simulink model "ErdMondBahn"  (R2014b)
settings: Solver=ode45  StartTime=0.0  StopTime=840000  RelTol=1e-3
libraries: simulink x1
settings Model: Creator=Florian  LastModifiedBy=Florian

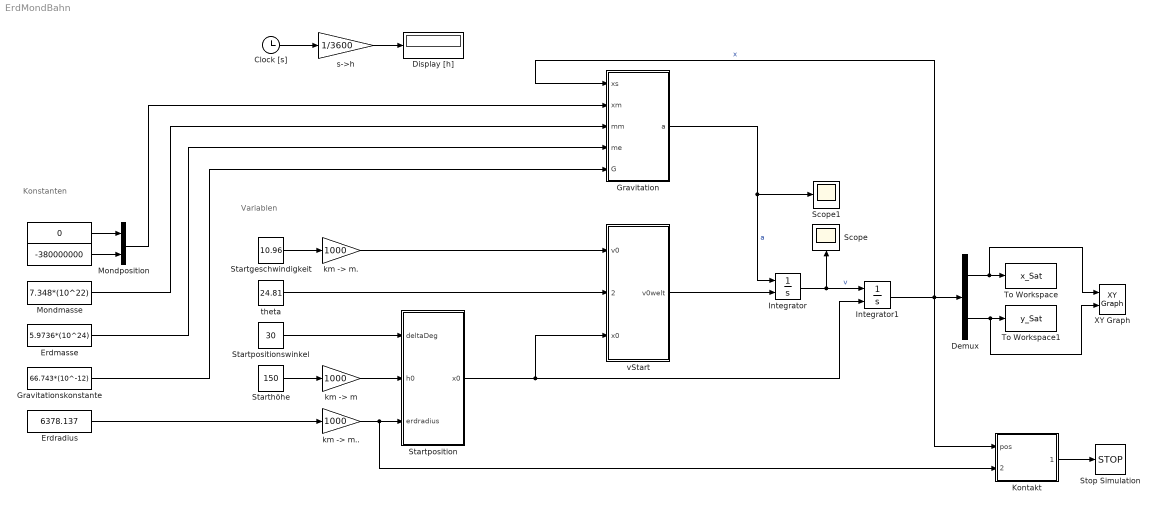
== system ErdMondBahn ==
  note: Konstanten
  note: Variablen
  "  " : Constant  Value=0
  "        " : Constant  Value=-380000000
  Clock [s] : Clock
  Demux : Demux  Outputs=2
  Display [h] : Display
  Erdmasse : Constant  Value=5.9736*(10^24)
  Erdradius : Constant  Value=6378.137
  Gravitation : MATLAB Function  TreatAsAtomicUnit=on
  Gravitationskonstante : Constant  Value=66.743*(10^-12)
  Integrator : Integrator  InitialConditionSource=external
  Integrator1 : Integrator  InitialConditionSource=external
  Kontakt : MATLAB Function  TreatAsAtomicUnit=on
  Mondmasse : Constant  Value=7.348*(10^22)
  Mondposition : Concatenate
  Scope : Scope
  Scope1 : Scope
  Startgeschwindigkeit : Constant  Value=10.96
  Starthöhe : Constant  Value=150
  Startposition : MATLAB Function  TreatAsAtomicUnit=on
  Startpositionswinkel : Constant  Value=30
  Stop Simulation : Stop
  To Workspace : ToWorkspace  VariableName=x_Sat  SampleTime=-1
  To Workspace1 : ToWorkspace  VariableName=y_Sat  SampleTime=-1
  XY Graph : simulink/Sinks/XY Graph  xmin=-22811188  xmax=22811188  ymin=-22811188  ymax=22811188  st=-1
  "km -> m" : Gain  Gain=1000
  "km -> m." : Gain  Gain=1000
  "km -> m.." : Gain  Gain=1000
  s->h : Gain  Gain=1/3600
  theta : Constant  Value=24.81
  vStart : MATLAB Function  TreatAsAtomicUnit=on
  wires:
  Erdradius/1 -> "km -> m.."/1
  Starthöhe/1 -> "km -> m"/1
  Startpositionswinkel/1 -> Startposition/1(deltaDeg)
  theta/1 -> vStart/2(thetaDeg)
  Startposition/1(x0) -> vStart/3(x0), Integrator1/2
  Kontakt/1(hasContact) -> Stop Simulation/1
  Clock [s]/1 -> s->h/1
  s->h/1 -> Display [h]/1
  Demux/1 -> XY Graph/1, To Workspace/1
  "km -> m"/1 -> Startposition/2(h0)
  "km -> m.."/1 -> Kontakt/2(erdradius), Startposition/3(erdradius)
  "km -> m."/1 -> vStart/1(v0)
  Gravitation/1(a) -> Integrator/1, Scope1/1  "a"
  Integrator/1 -> Integrator1/1, Scope/1  "v"
  Integrator1/1 -> Demux/1, Kontakt/1(pos), Gravitation/1(xs)  "x"
  Demux/2 -> XY Graph/2, To Workspace1/1
  Erdmasse/1 -> Gravitation/4(me)
  Gravitationskonstante/1 -> Gravitation/5(G)
  vStart/1(v0welt) -> Integrator/2
  Startgeschwindigkeit/1 -> "km -> m."/1
  Mondmasse/1 -> Gravitation/3(mm)
  "  "/1 -> Mondposition/1
  "        "/1 -> Mondposition/2
  Mondposition/1 -> Gravitation/2(xm)

== matlab function ErdMondBahn/vStart ==
  data: v0 input; thetaDeg input; x0 input; v0welt output
function v0welt = fcn(v0, thetaDeg, x0)
%-------------------------------------------------------------------------------------------------------
%Geben Sie eine EM-Funktion „vStart“ an,
%die aus den Parametern v0 ,  und der berechneten Startposition x0
%den Startgeschwindigkeitsvektor v0,Welt berechnet ( Anfangswert der Geschwindkt. in Weltkoordinaten).
%   Hinweis: - Einheitsvektoren in Tangential- und Normalenrichtung (n, t) aus x0 konstruieren,
%   - Tangential- und Normalkomponente der Startgeschwindigkeit (vt, vn) berechnen,
%   - aus n, t und (vt, vn) die Startgeschwindigkeit v0,Welt zusammenbauen.
%------------------------------------------------------------------------------------------------------


%Einheitsvektor von X0 (Normalenrichtung)
normalenrichtungX0 = x0 / norm(x0); %norm = Betrag -> x0/|x0|
%(Tangentialrichtung)
tangentialrichtungX0 = [normalenrichtungX0(2) ; -normalenrichtungX0(1)];  % [+;-]= im Uhrzeigersinn ; [-;+] = gegen Uhrzeigersinn


%Grad -> Bogenmaß
thetaBog = thetaDeg * (pi()/180);
%Tangential- und Normalkomponente der Startgeschwindigkeit
vt = cos(thetaBog) * v0;
vn = sin(thetaBog) * v0;


%Startgeschwindigkeit
v0welt = (norm(vt) * tangentialrichtungX0) + (norm(vn) * normalenrichtungX0);

== matlab function ErdMondBahn/Startposition ==
  data: deltaDeg input; x0 output; h0 input; erdradius input
function x0 = fcn(deltaDeg, h0, erdradius)
%-------------------------------------------------------------------------------------------------------
%Geben Sie eine Embedded-Matlab-(EM)-Funktion „Startposition“ an,
%die aus den Parametern delta(°), der Starthöhe h0 (km) sowie der Konstante „Erdradius“
%die Startposition x0 berechnet ( Anfangswert für die Position).
%------------------------------------------------------------------------------------------------------

%Grad -> Bogenmaß
deltaBog = deltaDeg* pi()/180;

hoehe = erdradius + h0;

x = cos(deltaBog)*(hoehe);
y = sin(deltaBog)*(hoehe);

x0 = [x;y];

== matlab function ErdMondBahn/Gravitation ==
  data: xs input; xm input; mm input; me input; a output; G input
function a = fcn(xs, xm, mm, me, G)
%-------------------------------------------------------------------------------------------------------
%Geben Sie eine EM-Funktion „Gravitation“ an,
%die aus der aktuellen Satellitenposition x,
%den auf den Satelliten wirkenden Gravitationsvektor errechnet (Hinweis: F=ma).
%-------------------------------------------------------------------------------------------------------


%xm= [0 ; -380000000];

%Entfernungen
abstandZurErde = norm(xs);    %Entfernung Erde-Satellit
abstandZumMond = norm(xm-xs); %Entfernung Mond-Satellit

%Einheitsvektor 
eES = (-xs / abstandZurErde); %Erdanziehungskraft (Erde auf Satellit) (e ES) [Folie 57]
eMS = ((xm-xs)/abstandZumMond); %Mondanziehungskraft (Mond auf Satellit) (e MS)

%Gravitationsbeschleunigung
a =G*( me/abstandZurErde^2 * eES + mm/abstandZumMond^2 * eMS);

== matlab function ErdMondBahn/Kontakt ==
  data: pos input; hasContact output; erdradius input
function hasContact = fcn(pos, erdradius)
%-------------------------------------------------------------------------------------------------------
%Geben Sie eine EM-Funktion „Kontakt“ an,
%die 0 ausgibt solange die Satellitenposition über der Erdoberfläche liegt, sonst 1.
%-------------------------------------------------------------------------------------------------------

if(norm(pos)<erdradius)
    hasContact = 1;
else
    hasContact = 0;
end;
